simulink model "Microgrid_W"  (R2020a)
settings: Solver=ode15s  StartTime=0  StopTime=1440*1  MaxStep=1  RelTol=1e-3
libraries: simulink x4214, powerlib x685, simulink_extras x28, Microgrid_Library x18, powerlib_meascontrol x12
(part 29 of 48)

== system Microgrid_W/House 4 W1/Light 1/D2 ==
  Add : Sum
  Clock1 : Clock
  Constant : Constant
  Constant1 : Constant  Value=0
  Gain : Gain  Gain=t
  Interval Test : simulink/Logic and Bit Operations/Interval Test  IntervalClosedRight=on  uplimit=K_L1_Off_1+86400  IntervalClosedLeft=on  lowlimit=K_L1_On_1+86400  OutDataTypeStr=boolean
  Interval Test1 : simulink/Logic and Bit Operations/Interval Test  IntervalClosedRight=on  uplimit=K_L1_Off_2+86400  IntervalClosedLeft=on  lowlimit=K_L1_On_2+86400  OutDataTypeStr=boolean
  Switch : Switch  Criteria=u2 > Threshold  Threshold=0.5
  Switch1 : Switch  Criteria=u2 > Threshold  Threshold=0.5
  Out1 : Outport  VectorParamsAs1DForOutWhenUnconnected=off
  wires:
  Interval Test/1 -> Switch/2
  Switch/1 -> Add/1
  Interval Test1/1 -> Switch1/2
  Add/1 -> Out1/1
  Constant1/1 -> Switch/3, Switch1/3
  Constant/1 -> Switch/1, Switch1/1
  Switch1/1 -> Add/2
  Gain/1 -> Interval Test1/1, Interval Test/1
  Clock1/1 -> Gain/1

== system Microgrid_W/House 4 W1/Light 1/D3 ==
  Add : Sum
  Clock1 : Clock
  Constant : Constant
  Constant1 : Constant  Value=0
  Gain : Gain  Gain=t
  Interval Test : simulink/Logic and Bit Operations/Interval Test  IntervalClosedRight=on  uplimit=K_L1_Off_1+86400*2  IntervalClosedLeft=on  lowlimit=K_L1_On_1+86400*2  OutDataTypeStr=boolean
  Interval Test1 : simulink/Logic and Bit Operations/Interval Test  IntervalClosedRight=on  uplimit=K_L1_Off_2+86400*2  IntervalClosedLeft=on  lowlimit=K_L1_On_2+86400*2  OutDataTypeStr=boolean
  Switch : Switch  Criteria=u2 > Threshold  Threshold=0.5
  Switch1 : Switch  Criteria=u2 > Threshold  Threshold=0.5
  Out1 : Outport  VectorParamsAs1DForOutWhenUnconnected=off
  wires:
  Gain/1 -> Interval Test/1, Interval Test1/1
  Switch1/1 -> Add/2
  Constant/1 -> Switch1/1, Switch/1
  Constant1/1 -> Switch1/3, Switch/3
  Add/1 -> Out1/1
  Interval Test1/1 -> Switch1/2
  Switch/1 -> Add/1
  Interval Test/1 -> Switch/2
  Clock1/1 -> Gain/1

== system Microgrid_W/House 4 W1/Light 1/D4 ==
  Add : Sum
  Clock : Clock
  Constant : Constant
  Constant1 : Constant  Value=0
  Gain : Gain  Gain=t
  Interval Test : simulink/Logic and Bit Operations/Interval Test  IntervalClosedRight=on  uplimit=K_L1_Off_1+86400*3  IntervalClosedLeft=on  lowlimit=K_L1_On_1+86400*3  OutDataTypeStr=boolean
  Interval Test1 : simulink/Logic and Bit Operations/Interval Test  IntervalClosedRight=on  uplimit=K_L1_Off_2+86400*3  IntervalClosedLeft=on  lowlimit=K_L1_On_2+86400*3  OutDataTypeStr=boolean
  Switch : Switch  Criteria=u2 > Threshold  Threshold=0.5
  Switch1 : Switch  Criteria=u2 > Threshold  Threshold=0.5
  Out1 : Outport  VectorParamsAs1DForOutWhenUnconnected=off
  wires:
  Interval Test/1 -> Switch/2
  Switch/1 -> Add/1
  Interval Test1/1 -> Switch1/2
  Add/1 -> Out1/1
  Constant1/1 -> Switch/3, Switch1/3
  Constant/1 -> Switch/1, Switch1/1
  Switch1/1 -> Add/2
  Gain/1 -> Interval Test1/1, Interval Test/1
  Clock/1 -> Gain/1

== system Microgrid_W/House 4 W1/Light 1/D5 ==
  Add : Sum
  Clock : Clock
  Constant : Constant
  Constant1 : Constant  Value=0
  Gain : Gain  Gain=t
  Interval Test : simulink/Logic and Bit Operations/Interval Test  IntervalClosedRight=on  uplimit=K_L1_Off_1+86400*4  IntervalClosedLeft=on  lowlimit=K_L1_On_1+86400*4  OutDataTypeStr=boolean
  Interval Test1 : simulink/Logic and Bit Operations/Interval Test  IntervalClosedRight=on  uplimit=K_L1_Off_2+86400*4  IntervalClosedLeft=on  lowlimit=K_L1_On_2+86400*4  OutDataTypeStr=boolean
  Switch : Switch  Criteria=u2 > Threshold  Threshold=0.5
  Switch1 : Switch  Criteria=u2 > Threshold  Threshold=0.5
  Out1 : Outport  VectorParamsAs1DForOutWhenUnconnected=off
  wires:
  Gain/1 -> Interval Test/1, Interval Test1/1
  Switch1/1 -> Add/2
  Constant/1 -> Switch1/1, Switch/1
  Constant1/1 -> Switch1/3, Switch/3
  Add/1 -> Out1/1
  Interval Test1/1 -> Switch1/2
  Switch/1 -> Add/1
  Interval Test/1 -> Switch/2
  Clock/1 -> Gain/1

== system Microgrid_W/House 4 W1/Light 1/D6 ==
  Add : Sum
  Clock : Clock
  Constant : Constant
  Constant1 : Constant  Value=0
  Gain : Gain  Gain=t
  Interval Test : simulink/Logic and Bit Operations/Interval Test  IntervalClosedRight=on  uplimit=K_L1_Off_1+86400*5  IntervalClosedLeft=on  lowlimit=K_L1_On_1+86400*5  OutDataTypeStr=boolean
  Interval Test1 : simulink/Logic and Bit Operations/Interval Test  IntervalClosedRight=on  uplimit=K_L1_Off_2+86400*5  IntervalClosedLeft=on  lowlimit=K_L1_On_2+86400*5  OutDataTypeStr=boolean
  Switch : Switch  Criteria=u2 > Threshold  Threshold=0.5
  Switch1 : Switch  Criteria=u2 > Threshold  Threshold=0.5
  Out1 : Outport  VectorParamsAs1DForOutWhenUnconnected=off
  wires:
  Interval Test/1 -> Switch/2
  Switch/1 -> Add/1
  Interval Test1/1 -> Switch1/2
  Add/1 -> Out1/1
  Constant1/1 -> Switch/3, Switch1/3
  Constant/1 -> Switch/1, Switch1/1
  Switch1/1 -> Add/2
  Gain/1 -> Interval Test1/1, Interval Test/1
  Clock/1 -> Gain/1

== system Microgrid_W/House 4 W1/Light 1/D7 ==
  Add : Sum
  Clock : Clock
  Constant : Constant
  Constant1 : Constant  Value=0
  Gain : Gain  Gain=t
  Interval Test : simulink/Logic and Bit Operations/Interval Test  IntervalClosedRight=on  uplimit=K_L1_Off_1+86400*6  IntervalClosedLeft=on  lowlimit=K_L1_On_1+86400*6  OutDataTypeStr=boolean
  Interval Test1 : simulink/Logic and Bit Operations/Interval Test  IntervalClosedRight=on  uplimit=K_L1_Off_2+86400*6  IntervalClosedLeft=on  lowlimit=K_L1_On_2+86400*6  OutDataTypeStr=boolean
  Switch : Switch  Criteria=u2 > Threshold  Threshold=0.5
  Switch1 : Switch  Criteria=u2 > Threshold  Threshold=0.5
  Out1 : Outport  VectorParamsAs1DForOutWhenUnconnected=off
  wires:
  Gain/1 -> Interval Test/1, Interval Test1/1
  Switch1/1 -> Add/2
  Constant/1 -> Switch1/1, Switch/1
  Constant1/1 -> Switch1/3, Switch/3
  Add/1 -> Out1/1
  Interval Test1/1 -> Switch1/2
  Switch/1 -> Add/1
  Interval Test/1 -> Switch/2
  Clock/1 -> Gain/1

== system Microgrid_W/House 4 W1/Light 2/D1 ==
  Clock : Clock
  Constant : Constant
  Constant1 : Constant  Value=0
  Gain : Gain  Gain=t
  Interval Test : simulink/Logic and Bit Operations/Interval Test  IntervalClosedRight=on  uplimit=K_L2_Off_1  IntervalClosedLeft=on  lowlimit=K_L2_On_1  OutDataTypeStr=boolean
  Switch : Switch  Criteria=u2 > Threshold  Threshold=0.5
  Out1 : Outport  VectorParamsAs1DForOutWhenUnconnected=off
  wires:
  Interval Test/1 -> Switch/2
  Switch/1 -> Out1/1
  Constant1/1 -> Switch/3
  Constant/1 -> Switch/1
  Gain/1 -> Interval Test/1
  Clock/1 -> Gain/1

== system Microgrid_W/House 4 W1/Light 2/D2 ==
  Clock : Clock
  Constant : Constant
  Constant1 : Constant  Value=0
  Gain : Gain  Gain=t
  Interval Test : simulink/Logic and Bit Operations/Interval Test  IntervalClosedRight=on  uplimit=K_L2_Off_1+86400  IntervalClosedLeft=on  lowlimit=K_L2_On_1+86400  OutDataTypeStr=boolean
  Switch : Switch  Criteria=u2 > Threshold  Threshold=0.5
  Out1 : Outport  VectorParamsAs1DForOutWhenUnconnected=off
  wires:
  Gain/1 -> Interval Test/1
  Constant/1 -> Switch/1
  Constant1/1 -> Switch/3
  Switch/1 -> Out1/1
  Interval Test/1 -> Switch/2
  Clock/1 -> Gain/1

== system Microgrid_W/House 4 W1/Light 2/D3 ==
  Clock : Clock
  Constant : Constant
  Constant1 : Constant  Value=0
  Gain : Gain  Gain=t
  Interval Test : simulink/Logic and Bit Operations/Interval Test  IntervalClosedRight=on  uplimit=K_L2_Off_1+86400*2  IntervalClosedLeft=on  lowlimit=K_L2_On_1+86400*2  OutDataTypeStr=boolean
  Switch : Switch  Criteria=u2 > Threshold  Threshold=0.5
  Out1 : Outport  VectorParamsAs1DForOutWhenUnconnected=off
  wires:
  Interval Test/1 -> Switch/2
  Switch/1 -> Out1/1
  Constant1/1 -> Switch/3
  Constant/1 -> Switch/1
  Gain/1 -> Interval Test/1
  Clock/1 -> Gain/1

== system Microgrid_W/House 4 W1/Light 2/D4 ==
  Clock : Clock
  Constant : Constant
  Constant1 : Constant  Value=0
  Gain : Gain  Gain=t
  Interval Test : simulink/Logic and Bit Operations/Interval Test  IntervalClosedRight=on  uplimit=K_L2_Off_1+86400*3  IntervalClosedLeft=on  lowlimit=K_L2_On_1+86400*3  OutDataTypeStr=boolean
  Switch : Switch  Criteria=u2 > Threshold  Threshold=0.5
  Out1 : Outport  VectorParamsAs1DForOutWhenUnconnected=off
  wires:
  Gain/1 -> Interval Test/1
  Constant/1 -> Switch/1
  Constant1/1 -> Switch/3
  Switch/1 -> Out1/1
  Interval Test/1 -> Switch/2
  Clock/1 -> Gain/1

== system Microgrid_W/House 4 W1/Light 2/D5 ==
  Clock : Clock
  Constant : Constant
  Constant1 : Constant  Value=0
  Gain : Gain  Gain=t
  Interval Test : simulink/Logic and Bit Operations/Interval Test  IntervalClosedRight=on  uplimit=K_L2_Off_1+86400*4  IntervalClosedLeft=on  lowlimit=K_L2_On_1+86400*4  OutDataTypeStr=boolean
  Switch : Switch  Criteria=u2 > Threshold  Threshold=0.5
  Out1 : Outport  VectorParamsAs1DForOutWhenUnconnected=off
  wires:
  Interval Test/1 -> Switch/2
  Switch/1 -> Out1/1
  Constant1/1 -> Switch/3
  Constant/1 -> Switch/1
  Gain/1 -> Interval Test/1
  Clock/1 -> Gain/1

== system Microgrid_W/House 4 W1/Light 2/D6 ==
  Clock : Clock
  Constant : Constant
  Constant1 : Constant  Value=0
  Gain : Gain  Gain=t
  Interval Test : simulink/Logic and Bit Operations/Interval Test  IntervalClosedRight=on  uplimit=K_L2_Off_1+86400*5  IntervalClosedLeft=on  lowlimit=K_L2_On_1+86400*5  OutDataTypeStr=boolean
  Switch : Switch  Criteria=u2 > Threshold  Threshold=0.5
  Out1 : Outport  VectorParamsAs1DForOutWhenUnconnected=off
  wires:
  Gain/1 -> Interval Test/1
  Constant/1 -> Switch/1
  Constant1/1 -> Switch/3
  Switch/1 -> Out1/1
  Interval Test/1 -> Switch/2
  Clock/1 -> Gain/1

== system Microgrid_W/House 4 W1/Light 2/D7 ==
  Clock : Clock
  Constant : Constant
  Constant1 : Constant  Value=0
  Gain : Gain  Gain=t
  Interval Test : simulink/Logic and Bit Operations/Interval Test  IntervalClosedRight=on  uplimit=K_L2_Off_1+86400*6  IntervalClosedLeft=on  lowlimit=K_L2_On_1+86400*6  OutDataTypeStr=boolean
  Switch : Switch  Criteria=u2 > Threshold  Threshold=0.5
  Out1 : Outport  VectorParamsAs1DForOutWhenUnconnected=off
  wires:
  Interval Test/1 -> Switch/2
  Switch/1 -> Out1/1
  Constant1/1 -> Switch/3
  Constant/1 -> Switch/1
  Gain/1 -> Interval Test/1
  Clock/1 -> Gain/1

== system Microgrid_W/House 4 W1/Light 3/D1 ==
  Add : Sum
  Clock : Clock
  Constant : Constant
  Constant1 : Constant  Value=0
  Gain : Gain  Gain=t
  Interval Test : simulink/Logic and Bit Operations/Interval Test  IntervalClosedRight=on  uplimit=K_L3_Off_1  IntervalClosedLeft=on  lowlimit=K_L3_On_1  OutDataTypeStr=boolean
  Interval Test1 : simulink/Logic and Bit Operations/Interval Test  IntervalClosedRight=on  uplimit=K_L3_Off_2  IntervalClosedLeft=on  lowlimit=K_L3_On_2  OutDataTypeStr=boolean
  Switch : Switch  Criteria=u2 > Threshold  Threshold=0.5
  Switch1 : Switch  Criteria=u2 > Threshold  Threshold=0.5
  Out1 : Outport  VectorParamsAs1DForOutWhenUnconnected=off
  wires:
  Interval Test/1 -> Switch/2
  Switch/1 -> Add/1
  Interval Test1/1 -> Switch1/2
  Add/1 -> Out1/1
  Constant1/1 -> Switch/3, Switch1/3
  Constant/1 -> Switch/1, Switch1/1
  Switch1/1 -> Add/2
  Gain/1 -> Interval Test1/1, Interval Test/1
  Clock/1 -> Gain/1

== system Microgrid_W/House 4 W1/Light 3/D2 ==
  Add : Sum
  Clock : Clock
  Constant : Constant
  Constant1 : Constant  Value=0
  Gain : Gain  Gain=t
  Interval Test : simulink/Logic and Bit Operations/Interval Test  IntervalClosedRight=on  uplimit=K_L3_Off_1+86400  IntervalClosedLeft=on  lowlimit=K_L3_On_1+86400  OutDataTypeStr=boolean
  Interval Test1 : simulink/Logic and Bit Operations/Interval Test  IntervalClosedRight=on  uplimit=K_L3_Off_2+86400  IntervalClosedLeft=on  lowlimit=K_L3_On_2+86400  OutDataTypeStr=boolean
  Switch : Switch  Criteria=u2 > Threshold  Threshold=0.5
  Switch1 : Switch  Criteria=u2 > Threshold  Threshold=0.5
  Out1 : Outport  VectorParamsAs1DForOutWhenUnconnected=off
  wires:
  Gain/1 -> Interval Test/1, Interval Test1/1
  Switch1/1 -> Add/2
  Constant/1 -> Switch1/1, Switch/1
  Constant1/1 -> Switch1/3, Switch/3
  Add/1 -> Out1/1
  Interval Test1/1 -> Switch1/2
  Switch/1 -> Add/1
  Interval Test/1 -> Switch/2
  Clock/1 -> Gain/1

== system Microgrid_W/House 4 W1/Light 3/D3 ==
  Add : Sum
  Clock : Clock
  Constant : Constant
  Constant1 : Constant  Value=0
  Gain : Gain  Gain=t
  Interval Test : simulink/Logic and Bit Operations/Interval Test  IntervalClosedRight=on  uplimit=K_L3_Off_1+86400*2  IntervalClosedLeft=on  lowlimit=K_L3_On_1+86400*2  OutDataTypeStr=boolean
  Interval Test1 : simulink/Logic and Bit Operations/Interval Test  IntervalClosedRight=on  uplimit=K_L3_Off_2+86400*2  IntervalClosedLeft=on  lowlimit=K_L3_On_2+86400*2  OutDataTypeStr=boolean
  Switch : Switch  Criteria=u2 > Threshold  Threshold=0.5
  Switch1 : Switch  Criteria=u2 > Threshold  Threshold=0.5
  Out1 : Outport  VectorParamsAs1DForOutWhenUnconnected=off
  wires:
  Interval Test/1 -> Switch/2
  Switch/1 -> Add/1
  Interval Test1/1 -> Switch1/2
  Add/1 -> Out1/1
  Constant1/1 -> Switch/3, Switch1/3
  Constant/1 -> Switch/1, Switch1/1
  Switch1/1 -> Add/2
  Gain/1 -> Interval Test1/1, Interval Test/1
  Clock/1 -> Gain/1

== system Microgrid_W/House 4 W1/Light 3/D4 ==
  Add : Sum
  Clock : Clock
  Constant : Constant
  Constant1 : Constant  Value=0
  Gain : Gain  Gain=t
  Interval Test : simulink/Logic and Bit Operations/Interval Test  IntervalClosedRight=on  uplimit=K_L3_Off_1+86400*3  IntervalClosedLeft=on  lowlimit=K_L3_On_1+86400*3  OutDataTypeStr=boolean
  Interval Test1 : simulink/Logic and Bit Operations/Interval Test  IntervalClosedRight=on  uplimit=K_L3_Off_2+86400*3  IntervalClosedLeft=on  lowlimit=K_L3_On_2+86400*3  OutDataTypeStr=boolean
  Switch : Switch  Criteria=u2 > Threshold  Threshold=0.5
  Switch1 : Switch  Criteria=u2 > Threshold  Threshold=0.5
  Out1 : Outport  VectorParamsAs1DForOutWhenUnconnected=off
  wires:
  Gain/1 -> Interval Test/1, Interval Test1/1
  Switch1/1 -> Add/2
  Constant/1 -> Switch1/1, Switch/1
  Constant1/1 -> Switch1/3, Switch/3
  Add/1 -> Out1/1
  Interval Test1/1 -> Switch1/2
  Switch/1 -> Add/1
  Interval Test/1 -> Switch/2
  Clock/1 -> Gain/1

== system Microgrid_W/House 4 W1/Light 3/D5 ==
  Add : Sum
  Clock : Clock
  Constant : Constant
  Constant1 : Constant  Value=0
  Gain : Gain  Gain=t
  Interval Test : simulink/Logic and Bit Operations/Interval Test  IntervalClosedRight=on  uplimit=K_L3_Off_1+86400*4  IntervalClosedLeft=on  lowlimit=K_L3_On_1+86400*4  OutDataTypeStr=boolean
  Interval Test1 : simulink/Logic and Bit Operations/Interval Test  IntervalClosedRight=on  uplimit=K_L3_Off_2+86400*4  IntervalClosedLeft=on  lowlimit=K_L3_On_2+86400*4  OutDataTypeStr=boolean
  Switch : Switch  Criteria=u2 > Threshold  Threshold=0.5
  Switch1 : Switch  Criteria=u2 > Threshold  Threshold=0.5
  Out1 : Outport  VectorParamsAs1DForOutWhenUnconnected=off
  wires:
  Interval Test/1 -> Switch/2
  Switch/1 -> Add/1
  Interval Test1/1 -> Switch1/2
  Add/1 -> Out1/1
  Constant1/1 -> Switch/3, Switch1/3
  Constant/1 -> Switch/1, Switch1/1
  Switch1/1 -> Add/2
  Gain/1 -> Interval Test1/1, Interval Test/1
  Clock/1 -> Gain/1

== system Microgrid_W/House 4 W1/Light 3/D6 ==
  Add : Sum
  Clock : Clock
  Constant : Constant
  Constant1 : Constant  Value=0
  Gain : Gain  Gain=t
  Interval Test : simulink/Logic and Bit Operations/Interval Test  IntervalClosedRight=on  uplimit=K_L3_Off_1+86400*5  IntervalClosedLeft=on  lowlimit=K_L3_On_1+86400*5  OutDataTypeStr=boolean
  Interval Test1 : simulink/Logic and Bit Operations/Interval Test  IntervalClosedRight=on  uplimit=K_L3_Off_2+86400*5  IntervalClosedLeft=on  lowlimit=K_L3_On_2+86400*5  OutDataTypeStr=boolean
  Switch : Switch  Criteria=u2 > Threshold  Threshold=0.5
  Switch1 : Switch  Criteria=u2 > Threshold  Threshold=0.5
  Out1 : Outport  VectorParamsAs1DForOutWhenUnconnected=off
  wires:
  ? -> Interval Test/1, Interval Test1/1
  Switch1/1 -> Add/2
  Constant/1 -> Switch1/1, Switch/1
  Constant1/1 -> Switch1/3, Switch/3
  Add/1 -> Out1/1
  Interval Test1/1 -> Switch1/2
  Switch/1 -> Add/1
  Interval Test/1 -> Switch/2
  Clock/1 -> Gain/1

== system Microgrid_W/House 4 W1/Light 3/D7 ==
  Add : Sum
  Clock : Clock
  Constant : Constant
  Constant1 : Constant  Value=0
  Gain : Gain  Gain=t
  Interval Test : simulink/Logic and Bit Operations/Interval Test  IntervalClosedRight=on  uplimit=K_L3_Off_1+86400*6  IntervalClosedLeft=on  lowlimit=K_L3_On_1+86400*6  OutDataTypeStr=boolean
  Interval Test1 : simulink/Logic and Bit Operations/Interval Test  IntervalClosedRight=on  uplimit=K_L3_Off_2+86400*6  IntervalClosedLeft=on  lowlimit=K_L3_On_2+86400*6  OutDataTypeStr=boolean
  Switch : Switch  Criteria=u2 > Threshold  Threshold=0.5
  Switch1 : Switch  Criteria=u2 > Threshold  Threshold=0.5
  Out1 : Outport  VectorParamsAs1DForOutWhenUnconnected=off
  wires:
  Interval Test/1 -> Switch/2
  Switch/1 -> Add/1
  Interval Test1/1 -> Switch1/2
  Add/1 -> Out1/1
  Constant1/1 -> Switch/3, Switch1/3
  Constant/1 -> Switch/1, Switch1/1
  Switch1/1 -> Add/2
  Gain/1 -> Interval Test1/1, Interval Test/1
  Clock/1 -> Gain/1

== system Microgrid_W/House 4 W1/Light 4/D1 ==
  Clock : Clock
  Constant : Constant
  Constant1 : Constant  Value=0
  Gain : Gain  Gain=t
  Interval Test : simulink/Logic and Bit Operations/Interval Test  IntervalClosedRight=on  uplimit=K_L4_Off_1  IntervalClosedLeft=on  lowlimit=K_L4_On_1  OutDataTypeStr=boolean
  Switch : Switch  Criteria=u2 > Threshold  Threshold=0.5
  Out1 : Outport  VectorParamsAs1DForOutWhenUnconnected=off
  wires:
  Interval Test/1 -> Switch/2
  Switch/1 -> Out1/1
  Constant1/1 -> Switch/3
  Constant/1 -> Switch/1
  Gain/1 -> Interval Test/1
  Clock/1 -> Gain/1

== system Microgrid_W/House 4 W1/Light 4/D2 ==
  Clock : Clock
  Constant : Constant
  Constant1 : Constant  Value=0
  Gain : Gain  Gain=t
  Interval Test : simulink/Logic and Bit Operations/Interval Test  IntervalClosedRight=on  uplimit=K_L4_Off_1+86400  IntervalClosedLeft=on  lowlimit=K_L4_On_1+86400  OutDataTypeStr=boolean
  Switch : Switch  Criteria=u2 > Threshold  Threshold=0.5
  Out1 : Outport  VectorParamsAs1DForOutWhenUnconnected=off
  wires:
  Gain/1 -> Interval Test/1
  Constant/1 -> Switch/1
  Constant1/1 -> Switch/3
  Switch/1 -> Out1/1
  Interval Test/1 -> Switch/2
  Clock/1 -> Gain/1

== system Microgrid_W/House 4 W1/Light 4/D3 ==
  Clock : Clock
  Constant : Constant
  Constant1 : Constant  Value=0
  Gain : Gain  Gain=t
  Interval Test : simulink/Logic and Bit Operations/Interval Test  IntervalClosedRight=on  uplimit=K_L4_Off_1+86400*2  IntervalClosedLeft=on  lowlimit=K_L4_On_1+86400*2  OutDataTypeStr=boolean
  Switch : Switch  Criteria=u2 > Threshold  Threshold=0.5
  Out1 : Outport  VectorParamsAs1DForOutWhenUnconnected=off
  wires:
  Interval Test/1 -> Switch/2
  Switch/1 -> Out1/1
  Constant1/1 -> Switch/3
  Constant/1 -> Switch/1
  Gain/1 -> Interval Test/1
  Clock/1 -> Gain/1

== system Microgrid_W/House 4 W1/Light 4/D4 ==
  Clock : Clock
  Constant : Constant
  Constant1 : Constant  Value=0
  Gain : Gain  Gain=t
  Interval Test : simulink/Logic and Bit Operations/Interval Test  IntervalClosedRight=on  uplimit=K_L4_Off_1+86400*3  IntervalClosedLeft=on  lowlimit=K_L4_On_1+86400*3  OutDataTypeStr=boolean
  Switch : Switch  Criteria=u2 > Threshold  Threshold=0.5
  Out1 : Outport  VectorParamsAs1DForOutWhenUnconnected=off
  wires:
  Gain/1 -> Interval Test/1
  Constant/1 -> Switch/1
  Constant1/1 -> Switch/3
  Switch/1 -> Out1/1
  Interval Test/1 -> Switch/2
  Clock/1 -> Gain/1

== system Microgrid_W/House 4 W1/Light 4/D5 ==
  Clock : Clock
  Constant : Constant
  Constant1 : Constant  Value=0
  Gain : Gain  Gain=t
  Interval Test : simulink/Logic and Bit Operations/Interval Test  IntervalClosedRight=on  uplimit=K_L4_Off_1+86400*4  IntervalClosedLeft=on  lowlimit=K_L4_On_1+86400*4  OutDataTypeStr=boolean
  Switch : Switch  Criteria=u2 > Threshold  Threshold=0.5
  Out1 : Outport  VectorParamsAs1DForOutWhenUnconnected=off
  wires:
  Interval Test/1 -> Switch/2
  Switch/1 -> Out1/1
  Constant1/1 -> Switch/3
  Constant/1 -> Switch/1
  Gain/1 -> Interval Test/1
  Clock/1 -> Gain/1

== system Microgrid_W/House 4 W1/Light 4/D6 ==
  Clock : Clock
  Constant : Constant
  Constant1 : Constant  Value=0
  Gain : Gain  Gain=t
  Interval Test : simulink/Logic and Bit Operations/Interval Test  IntervalClosedRight=on  uplimit=K_L4_Off_1+86400*5  IntervalClosedLeft=on  lowlimit=K_L4_On_1+86400*5  OutDataTypeStr=boolean
  Switch : Switch  Criteria=u2 > Threshold  Threshold=0.5
  Out1 : Outport  VectorParamsAs1DForOutWhenUnconnected=off
  wires:
  Gain/1 -> Interval Test/1
  Constant/1 -> Switch/1
  Constant1/1 -> Switch/3
  Switch/1 -> Out1/1
  Interval Test/1 -> Switch/2
  Clock/1 -> Gain/1

== system Microgrid_W/House 4 W1/Light 4/D7 ==
  Clock : Clock
  Constant : Constant
  Constant1 : Constant  Value=0
  Gain : Gain  Gain=t
  Interval Test : simulink/Logic and Bit Operations/Interval Test  IntervalClosedRight=on  uplimit=K_L4_Off_1+86400*6  IntervalClosedLeft=on  lowlimit=K_L4_On_1+86400*6  OutDataTypeStr=boolean
  Switch : Switch  Criteria=u2 > Threshold  Threshold=0.5
  Out1 : Outport  VectorParamsAs1DForOutWhenUnconnected=off
  wires:
  Interval Test/1 -> Switch/2
  Switch/1 -> Out1/1
  Constant1/1 -> Switch/3
  Constant/1 -> Switch/1
  Gain/1 -> Interval Test/1
  Clock/1 -> Gain/1

== system Microgrid_W/House 4 W1/Light 5/D1 ==
  Add : Sum
  Clock : Clock
  Constant : Constant
  Constant1 : Constant  Value=0
  Gain : Gain  Gain=t
  Interval Test : simulink/Logic and Bit Operations/Interval Test  IntervalClosedRight=on  uplimit=K_L5_Off_1  IntervalClosedLeft=on  lowlimit=K_L5_On_1  OutDataTypeStr=boolean
  Interval Test1 : simulink/Logic and Bit Operations/Interval Test  IntervalClosedRight=on  uplimit=K_L5_Off_2  IntervalClosedLeft=on  lowlimit=K_L5_On_2  OutDataTypeStr=boolean
  Switch : Switch  Criteria=u2 > Threshold  Threshold=0.5
  Switch1 : Switch  Criteria=u2 > Threshold  Threshold=0.5
  Out1 : Outport  VectorParamsAs1DForOutWhenUnconnected=off
  wires:
  Gain/1 -> Interval Test/1, Interval Test1/1
  Switch1/1 -> Add/2
  Constant/1 -> Switch1/1, Switch/1
  Constant1/1 -> Switch1/3, Switch/3
  Add/1 -> Out1/1
  Interval Test1/1 -> Switch1/2
  Switch/1 -> Add/1
  Interval Test/1 -> Switch/2
  Clock/1 -> Gain/1

== system Microgrid_W/House 4 W1/Light 5/D2 ==
  Add : Sum
  Clock : Clock
  Constant : Constant
  Constant1 : Constant  Value=0
  Gain : Gain  Gain=t
  Interval Test : simulink/Logic and Bit Operations/Interval Test  IntervalClosedRight=on  uplimit=K_L5_Off_1+86400  IntervalClosedLeft=on  lowlimit=K_L5_On_1+86400  OutDataTypeStr=boolean
  Interval Test1 : simulink/Logic and Bit Operations/Interval Test  IntervalClosedRight=on  uplimit=K_L5_Off_2+86400  IntervalClosedLeft=on  lowlimit=K_L5_On_2+86400  OutDataTypeStr=boolean
  Switch : Switch  Criteria=u2 > Threshold  Threshold=0.5
  Switch1 : Switch  Criteria=u2 > Threshold  Threshold=0.5
  Out1 : Outport  VectorParamsAs1DForOutWhenUnconnected=off
  wires:
  Interval Test/1 -> Switch/2
  Switch/1 -> Add/1
  Interval Test1/1 -> Switch1/2
  Add/1 -> Out1/1
  Constant1/1 -> Switch/3, Switch1/3
  Constant/1 -> Switch/1, Switch1/1
  Switch1/1 -> Add/2
  Gain/1 -> Interval Test1/1, Interval Test/1
  Clock/1 -> Gain/1

== system Microgrid_W/House 4 W1/Light 5/D3 ==
  Add : Sum
  Clock : Clock
  Constant : Constant
  Constant1 : Constant  Value=0
  Gain : Gain  Gain=t
  Interval Test : simulink/Logic and Bit Operations/Interval Test  IntervalClosedRight=on  uplimit=K_L5_Off_1+86400*2  IntervalClosedLeft=on  lowlimit=K_L5_On_1+86400*2  OutDataTypeStr=boolean
  Interval Test1 : simulink/Logic and Bit Operations/Interval Test  IntervalClosedRight=on  uplimit=K_L5_Off_2+86400*2  IntervalClosedLeft=on  lowlimit=K_L5_On_2+86400*2  OutDataTypeStr=boolean
  Switch : Switch  Criteria=u2 > Threshold  Threshold=0.5
  Switch1 : Switch  Criteria=u2 > Threshold  Threshold=0.5
  Out1 : Outport  VectorParamsAs1DForOutWhenUnconnected=off
  wires:
  Gain/1 -> Interval Test/1, Interval Test1/1
  Switch1/1 -> Add/2
  Constant/1 -> Switch1/1, Switch/1
  Constant1/1 -> Switch1/3, Switch/3
  Add/1 -> Out1/1
  Interval Test1/1 -> Switch1/2
  Switch/1 -> Add/1
  Interval Test/1 -> Switch/2
  Clock/1 -> Gain/1

== system Microgrid_W/House 4 W1/Light 5/D4 ==
  Add : Sum
  Clock : Clock
  Constant : Constant
  Constant1 : Constant  Value=0
  Gain : Gain  Gain=t
  Interval Test : simulink/Logic and Bit Operations/Interval Test  IntervalClosedRight=on  uplimit=K_L5_Off_1+86400*3  IntervalClosedLeft=on  lowlimit=K_L5_On_1+86400*3  OutDataTypeStr=boolean
  Interval Test1 : simulink/Logic and Bit Operations/Interval Test  IntervalClosedRight=on  uplimit=K_L5_Off_2+86400*3  IntervalClosedLeft=on  lowlimit=K_L5_On_2+86400*3  OutDataTypeStr=boolean
  Switch : Switch  Criteria=u2 > Threshold  Threshold=0.5
  Switch1 : Switch  Criteria=u2 > Threshold  Threshold=0.5
  Out1 : Outport  VectorParamsAs1DForOutWhenUnconnected=off
  wires:
  Interval Test/1 -> Switch/2
  Switch/1 -> Add/1
  Interval Test1/1 -> Switch1/2
  Add/1 -> Out1/1
  Constant1/1 -> Switch/3, Switch1/3
  Constant/1 -> Switch/1, Switch1/1
  Switch1/1 -> Add/2
  Gain/1 -> Interval Test1/1, Interval Test/1
  Clock/1 -> Gain/1

== system Microgrid_W/House 4 W1/Light 5/D5 ==
  Add : Sum
  Clock : Clock
  Constant : Constant
  Constant1 : Constant  Value=0
  Gain : Gain  Gain=t
  Interval Test : simulink/Logic and Bit Operations/Interval Test  IntervalClosedRight=on  uplimit=K_L5_Off_1+86400*4  IntervalClosedLeft=on  lowlimit=K_L5_On_1+86400*4  OutDataTypeStr=boolean
  Interval Test1 : simulink/Logic and Bit Operations/Interval Test  IntervalClosedRight=on  uplimit=K_L5_Off_2+86400*4  IntervalClosedLeft=on  lowlimit=K_L5_On_2+86400*4  OutDataTypeStr=boolean
  Switch : Switch  Criteria=u2 > Threshold  Threshold=0.5
  Switch1 : Switch  Criteria=u2 > Threshold  Threshold=0.5
  Out1 : Outport  VectorParamsAs1DForOutWhenUnconnected=off
  wires:
  Gain/1 -> Interval Test/1, Interval Test1/1
  Switch1/1 -> Add/2
  Constant/1 -> Switch1/1, Switch/1
  Constant1/1 -> Switch1/3, Switch/3
  Add/1 -> Out1/1
  Interval Test1/1 -> Switch1/2
  Switch/1 -> Add/1
  Interval Test/1 -> Switch/2
  Clock/1 -> Gain/1

== system Microgrid_W/House 4 W1/Light 5/D6 ==
  Add : Sum
  Clock : Clock
  Constant : Constant
  Constant1 : Constant  Value=0
  Gain : Gain  Gain=t
  Interval Test : simulink/Logic and Bit Operations/Interval Test  IntervalClosedRight=on  uplimit=K_L5_Off_1+86400*5  IntervalClosedLeft=on  lowlimit=K_L5_On_1+86400*5  OutDataTypeStr=boolean
  Interval Test1 : simulink/Logic and Bit Operations/Interval Test  IntervalClosedRight=on  uplimit=K_L5_Off_2+86400*5  IntervalClosedLeft=on  lowlimit=K_L5_On_2+86400*5  OutDataTypeStr=boolean
  Switch : Switch  Criteria=u2 > Threshold  Threshold=0.5
  Switch1 : Switch  Criteria=u2 > Threshold  Threshold=0.5
  Out1 : Outport  VectorParamsAs1DForOutWhenUnconnected=off
  wires:
  Interval Test/1 -> Switch/2
  Switch/1 -> Add/1
  Interval Test1/1 -> Switch1/2
  Add/1 -> Out1/1
  Constant1/1 -> Switch/3, Switch1/3
  Constant/1 -> Switch/1, Switch1/1
  Switch1/1 -> Add/2
  Gain/1 -> Interval Test1/1, Interval Test/1
  Clock/1 -> Gain/1

== system Microgrid_W/House 4 W1/Light 5/D7 ==
  Add : Sum
  Clock : Clock
  Constant : Constant
  Constant1 : Constant  Value=0
  Gain : Gain  Gain=t
  Interval Test : simulink/Logic and Bit Operations/Interval Test  IntervalClosedRight=on  uplimit=K_L5_Off_1+86400*6  IntervalClosedLeft=on  lowlimit=K_L5_On_1+86400*6  OutDataTypeStr=boolean
  Interval Test1 : simulink/Logic and Bit Operations/Interval Test  IntervalClosedRight=on  uplimit=K_L5_Off_2+86400*6  IntervalClosedLeft=on  lowlimit=K_L5_On_2+86400*6  OutDataTypeStr=boolean
  Switch : Switch  Criteria=u2 > Threshold  Threshold=0.5
  Switch1 : Switch  Criteria=u2 > Threshold  Threshold=0.5
  Out1 : Outport  VectorParamsAs1DForOutWhenUnconnected=off
  wires:
  Gain/1 -> Interval Test/1, Interval Test1/1
  Switch1/1 -> Add/2
  Constant/1 -> Switch1/1, Switch/1
  Constant1/1 -> Switch1/3, Switch/3
  Add/1 -> Out1/1
  Interval Test1/1 -> Switch1/2
  Switch/1 -> Add/1
  Interval Test/1 -> Switch/2
  Clock/1 -> Gain/1

== system Microgrid_W/House 4 W1/Light 6/D1 ==
  Clock : Clock
  Constant : Constant
  Constant1 : Constant  Value=0
  Gain : Gain  Gain=t
  Interval Test : simulink/Logic and Bit Operations/Interval Test  IntervalClosedRight=on  uplimit=K_L6_Off_1  IntervalClosedLeft=on  lowlimit=K_L6_On_1  OutDataTypeStr=boolean
  Switch : Switch  Criteria=u2 > Threshold  Threshold=0.5
  Out1 : Outport  VectorParamsAs1DForOutWhenUnconnected=off
  wires:
  Interval Test/1 -> Switch/2
  Switch/1 -> Out1/1
  Constant1/1 -> Switch/3
  Constant/1 -> Switch/1
  Gain/1 -> Interval Test/1
  Clock/1 -> Gain/1

== system Microgrid_W/House 4 W1/Light 6/D2 ==
  Clock : Clock
  Constant : Constant
  Constant1 : Constant  Value=0
  Gain : Gain  Gain=t
  Interval Test : simulink/Logic and Bit Operations/Interval Test  IntervalClosedRight=on  uplimit=K_L6_Off_1+86400  IntervalClosedLeft=on  lowlimit=K_L6_On_1+86400  OutDataTypeStr=boolean
  Switch : Switch  Criteria=u2 > Threshold  Threshold=0.5
  Out1 : Outport  VectorParamsAs1DForOutWhenUnconnected=off
  wires:
  Gain/1 -> Interval Test/1
  Constant/1 -> Switch/1
  Constant1/1 -> Switch/3
  Switch/1 -> Out1/1
  Interval Test/1 -> Switch/2
  Clock/1 -> Gain/1

== system Microgrid_W/House 4 W1/Light 6/D3 ==
  Clock : Clock
  Constant : Constant
  Constant1 : Constant  Value=0
  Gain : Gain  Gain=t
  Interval Test : simulink/Logic and Bit Operations/Interval Test  IntervalClosedRight=on  uplimit=K_L6_Off_1+86400*2  IntervalClosedLeft=on  lowlimit=K_L6_On_1+86400*2  OutDataTypeStr=boolean
  Switch : Switch  Criteria=u2 > Threshold  Threshold=0.5
  Out1 : Outport  VectorParamsAs1DForOutWhenUnconnected=off
  wires:
  Interval Test/1 -> Switch/2
  Switch/1 -> Out1/1
  Constant1/1 -> Switch/3
  Constant/1 -> Switch/1
  Gain/1 -> Interval Test/1
  Clock/1 -> Gain/1

== system Microgrid_W/House 4 W1/Light 6/D4 ==
  Clock : Clock
  Constant : Constant
  Constant1 : Constant  Value=0
  Gain : Gain  Gain=t
  Interval Test : simulink/Logic and Bit Operations/Interval Test  IntervalClosedRight=on  uplimit=K_L6_Off_1+86400*3  IntervalClosedLeft=on  lowlimit=K_L6_On_1+86400*3  OutDataTypeStr=boolean
  Switch : Switch  Criteria=u2 > Threshold  Threshold=0.5
  Out1 : Outport  VectorParamsAs1DForOutWhenUnconnected=off
  wires:
  Gain/1 -> Interval Test/1
  Constant/1 -> Switch/1
  Constant1/1 -> Switch/3
  Switch/1 -> Out1/1
  Interval Test/1 -> Switch/2
  Clock/1 -> Gain/1

== system Microgrid_W/House 4 W1/Light 6/D5 ==
  Clock : Clock
  Constant : Constant
  Constant1 : Constant  Value=0
  Gain : Gain  Gain=t
  Interval Test : simulink/Logic and Bit Operations/Interval Test  IntervalClosedRight=on  uplimit=K_L6_Off_1+86400*4  IntervalClosedLeft=on  lowlimit=K_L6_On_1+86400*4  OutDataTypeStr=boolean
  Switch : Switch  Criteria=u2 > Threshold  Threshold=0.5
  Out1 : Outport  VectorParamsAs1DForOutWhenUnconnected=off
  wires:
  Interval Test/1 -> Switch/2
  Switch/1 -> Out1/1
  Constant1/1 -> Switch/3
  Constant/1 -> Switch/1
  Gain/1 -> Interval Test/1
  Clock/1 -> Gain/1

== system Microgrid_W/House 4 W1/Light 6/D6 ==
  Clock : Clock
  Constant : Constant
  Constant1 : Constant  Value=0
  Gain : Gain  Gain=t
  Interval Test : simulink/Logic and Bit Operations/Interval Test  IntervalClosedRight=on  uplimit=K_L6_Off_1+86400*5  IntervalClosedLeft=on  lowlimit=K_L6_On_1+86400*5  OutDataTypeStr=boolean
  Switch : Switch  Criteria=u2 > Threshold  Threshold=0.5
  Out1 : Outport  VectorParamsAs1DForOutWhenUnconnected=off
  wires:
  Gain/1 -> Interval Test/1
  Constant/1 -> Switch/1
  Constant1/1 -> Switch/3
  Switch/1 -> Out1/1
  Interval Test/1 -> Switch/2
  Clock/1 -> Gain/1

== system Microgrid_W/House 4 W1/Light 6/D7 ==
  Clock : Clock
  Constant : Constant
  Constant1 : Constant  Value=0
  Gain : Gain  Gain=t
  Interval Test : simulink/Logic and Bit Operations/Interval Test  IntervalClosedRight=on  uplimit=K_L6_Off_1+86400*6  IntervalClosedLeft=on  lowlimit=K_L6_On_1+86400*6  OutDataTypeStr=boolean
  Switch : Switch  Criteria=u2 > Threshold  Threshold=0.5
  Out1 : Outport  VectorParamsAs1DForOutWhenUnconnected=off
  wires:
  Interval Test/1 -> Switch/2
  Switch/1 -> Out1/1
  Constant1/1 -> Switch/3
  Constant/1 -> Switch/1
  Gain/1 -> Interval Test/1
  Clock/1 -> Gain/1

== system Microgrid_W/House 4 W1/Oven/D1 ==
  Clock : Clock
  Constant : Constant
  Constant1 : Constant  Value=0
  Gain : Gain  Gain=t
  Interval Test : simulink/Logic and Bit Operations/Interval Test  IntervalClosedRight=on  uplimit=Oven_Off_1  IntervalClosedLeft=on  lowlimit=Oven_On_1  OutDataTypeStr=boolean
  Switch : Switch  Criteria=u2 > Threshold  Threshold=0.5
  Out1 : Outport  VectorParamsAs1DForOutWhenUnconnected=off
  wires:
  Interval Test/1 -> Switch/2
  Switch/1 -> Out1/1
  Constant1/1 -> Switch/3
  Constant/1 -> Switch/1
  Gain/1 -> Interval Test/1
  Clock/1 -> Gain/1

== system Microgrid_W/House 4 W1/Oven/D2 ==
  Clock : Clock
  Constant : Constant
  Constant1 : Constant  Value=0
  Gain : Gain  Gain=t
  Interval Test : simulink/Logic and Bit Operations/Interval Test  IntervalClosedRight=on  uplimit=Oven_Off_1+86400  IntervalClosedLeft=on  lowlimit=Oven_On_1+86400  OutDataTypeStr=boolean
  Switch : Switch  Criteria=u2 > Threshold  Threshold=0.5
  Out1 : Outport  VectorParamsAs1DForOutWhenUnconnected=off
  wires:
  Gain/1 -> Interval Test/1
  Constant/1 -> Switch/1
  Constant1/1 -> Switch/3
  Switch/1 -> Out1/1
  Interval Test/1 -> Switch/2
  Clock/1 -> Gain/1

== system Microgrid_W/House 4 W1/Oven/D3 ==
  Clock : Clock
  Constant : Constant
  Constant1 : Constant  Value=0
  Gain : Gain  Gain=t
  Interval Test : simulink/Logic and Bit Operations/Interval Test  IntervalClosedRight=on  uplimit=Oven_Off_1+86400*2  IntervalClosedLeft=on  lowlimit=Oven_On_1+86400*2  OutDataTypeStr=boolean
  Switch : Switch  Criteria=u2 > Threshold  Threshold=0.5
  Out1 : Outport  VectorParamsAs1DForOutWhenUnconnected=off
  wires:
  Interval Test/1 -> Switch/2
  Switch/1 -> Out1/1
  Constant1/1 -> Switch/3
  Constant/1 -> Switch/1
  Gain/1 -> Interval Test/1
  Clock/1 -> Gain/1

== system Microgrid_W/House 4 W1/Oven/D4 ==
  Clock : Clock
  Constant : Constant
  Constant1 : Constant  Value=0
  Gain : Gain  Gain=t
  Interval Test : simulink/Logic and Bit Operations/Interval Test  IntervalClosedRight=on  uplimit=Oven_Off_1+86400*3  IntervalClosedLeft=on  lowlimit=Oven_On_1+86400*3  OutDataTypeStr=boolean
  Switch : Switch  Criteria=u2 > Threshold  Threshold=0.5
  Out1 : Outport  VectorParamsAs1DForOutWhenUnconnected=off
  wires:
  Gain/1 -> Interval Test/1
  Constant/1 -> Switch/1
  Constant1/1 -> Switch/3
  Switch/1 -> Out1/1
  Interval Test/1 -> Switch/2
  Clock/1 -> Gain/1

== system Microgrid_W/House 4 W1/Oven/D5 ==
  Clock : Clock
  Constant : Constant
  Constant1 : Constant  Value=0
  Gain : Gain  Gain=t
  Interval Test : simulink/Logic and Bit Operations/Interval Test  IntervalClosedRight=on  uplimit=Oven_Off_1+86400*4  IntervalClosedLeft=on  lowlimit=Oven_On_1+86400*4  OutDataTypeStr=boolean
  Switch : Switch  Criteria=u2 > Threshold  Threshold=0.5
  Out1 : Outport  VectorParamsAs1DForOutWhenUnconnected=off
  wires:
  Interval Test/1 -> Switch/2
  Switch/1 -> Out1/1
  Constant1/1 -> Switch/3
  Constant/1 -> Switch/1
  Gain/1 -> Interval Test/1
  Clock/1 -> Gain/1

== system Microgrid_W/House 4 W1/Oven/D6 ==
  Clock : Clock
  Constant : Constant
  Constant1 : Constant  Value=0
  Gain : Gain  Gain=t
  Interval Test : simulink/Logic and Bit Operations/Interval Test  IntervalClosedRight=on  uplimit=Oven_Off_1+86400*5  IntervalClosedLeft=on  lowlimit=Oven_On_1+86400*5  OutDataTypeStr=boolean
  Switch : Switch  Criteria=u2 > Threshold  Threshold=0.5
  Out1 : Outport  VectorParamsAs1DForOutWhenUnconnected=off
  wires:
  Gain/1 -> Interval Test/1
  Constant/1 -> Switch/1
  Constant1/1 -> Switch/3
  Switch/1 -> Out1/1
  Interval Test/1 -> Switch/2
  Clock/1 -> Gain/1

== system Microgrid_W/House 4 W1/Oven/D7 ==
  Clock : Clock
  Constant : Constant
  Constant1 : Constant  Value=0
  Gain : Gain  Gain=t
  Interval Test : simulink/Logic and Bit Operations/Interval Test  IntervalClosedRight=on  uplimit=Oven_Off_1+86400*6  IntervalClosedLeft=on  lowlimit=Oven_On_1+86400*6  OutDataTypeStr=boolean
  Switch : Switch  Criteria=u2 > Threshold  Threshold=0.5
  Out1 : Outport  VectorParamsAs1DForOutWhenUnconnected=off
  wires:
  Interval Test/1 -> Switch/2
  Switch/1 -> Out1/1
  Constant1/1 -> Switch/3
  Constant/1 -> Switch/1
  Gain/1 -> Interval Test/1
  Clock/1 -> Gain/1

== system Microgrid_W/House 4 W1/Phone_Charger/D1 ==
  Add : Sum
  Clock : Clock
  Constant : Constant
  Constant1 : Constant  Value=0
  Gain : Gain  Gain=t
  Interval Test : simulink/Logic and Bit Operations/Interval Test  IntervalClosedRight=on  uplimit=Phone_C_1_Off_a  IntervalClosedLeft=on  lowlimit=Phone_C_1_On_a  OutDataTypeStr=boolean
  Interval Test1 : simulink/Logic and Bit Operations/Interval Test  IntervalClosedRight=on  uplimit=Phone_C_1_Off_b  IntervalClosedLeft=on  lowlimit=Phone_C_1_On_b  OutDataTypeStr=boolean
  Switch : Switch  Criteria=u2 > Threshold  Threshold=0.5
  Switch1 : Switch  Criteria=u2 > Threshold  Threshold=0.5
  Out1 : Outport  VectorParamsAs1DForOutWhenUnconnected=off
  wires:
  Gain/1 -> Interval Test/1, Interval Test1/1
  Switch1/1 -> Add/2
  Constant/1 -> Switch1/1, Switch/1
  Constant1/1 -> Switch1/3, Switch/3
  Add/1 -> Out1/1
  Interval Test1/1 -> Switch1/2
  Switch/1 -> Add/1
  Interval Test/1 -> Switch/2
  Clock/1 -> Gain/1

== system Microgrid_W/House 4 W1/Phone_Charger/D10 ==
  Add : Sum
  Clock : Clock
  Constant : Constant
  Constant1 : Constant  Value=0
  Gain : Gain  Gain=t
  Interval Test : simulink/Logic and Bit Operations/Interval Test  IntervalClosedRight=on  uplimit=Phone_C_2_Off_a+86400*2  IntervalClosedLeft=on  lowlimit=Phone_C_2_On_a+86400*2  OutDataTypeStr=boolean
  Interval Test1 : simulink/Logic and Bit Operations/Interval Test  IntervalClosedRight=on  uplimit=Phone_C_2_Off_b+86400*2  IntervalClosedLeft=on  lowlimit=Phone_C_2_On_b+86400*2  OutDataTypeStr=boolean
  Switch : Switch  Criteria=u2 > Threshold  Threshold=0.5
  Switch1 : Switch  Criteria=u2 > Threshold  Threshold=0.5
  Out1 : Outport  VectorParamsAs1DForOutWhenUnconnected=off
  wires:
  Interval Test/1 -> Switch/2
  Switch/1 -> Add/1
  Interval Test1/1 -> Switch1/2
  Add/1 -> Out1/1
  Constant1/1 -> Switch/3, Switch1/3
  Constant/1 -> Switch/1, Switch1/1
  Switch1/1 -> Add/2
  Gain/1 -> Interval Test1/1, Interval Test/1
  Clock/1 -> Gain/1

== system Microgrid_W/House 4 W1/Phone_Charger/D11 ==
  Add : Sum
  Clock : Clock
  Constant : Constant
  Constant1 : Constant  Value=0
  Gain : Gain  Gain=t
  Interval Test : simulink/Logic and Bit Operations/Interval Test  IntervalClosedRight=on  uplimit=Phone_C_2_Off_a+86400*3  IntervalClosedLeft=on  lowlimit=Phone_C_2_On_a+86400*3  OutDataTypeStr=boolean
  Interval Test1 : simulink/Logic and Bit Operations/Interval Test  IntervalClosedRight=on  uplimit=Phone_C_2_Off_b+86400*3  IntervalClosedLeft=on  lowlimit=Phone_C_2_On_b+86400*3  OutDataTypeStr=boolean
  Switch : Switch  Criteria=u2 > Threshold  Threshold=0.5
  Switch1 : Switch  Criteria=u2 > Threshold  Threshold=0.5
  Out1 : Outport  VectorParamsAs1DForOutWhenUnconnected=off
  wires:
  Gain/1 -> Interval Test/1, Interval Test1/1
  Switch1/1 -> Add/2
  Constant/1 -> Switch1/1, Switch/1
  Constant1/1 -> Switch1/3, Switch/3
  Add/1 -> Out1/1
  Interval Test1/1 -> Switch1/2
  Switch/1 -> Add/1
  Interval Test/1 -> Switch/2
  Clock/1 -> Gain/1

== system Microgrid_W/House 4 W1/Phone_Charger/D12 ==
  Add : Sum
  Clock : Clock
  Constant : Constant
  Constant1 : Constant  Value=0
  Gain : Gain  Gain=t
  Interval Test : simulink/Logic and Bit Operations/Interval Test  IntervalClosedRight=on  uplimit=Phone_C_2_Off_a+86400*4  IntervalClosedLeft=on  lowlimit=Phone_C_2_On_a+86400*4  OutDataTypeStr=boolean
  Interval Test1 : simulink/Logic and Bit Operations/Interval Test  IntervalClosedRight=on  uplimit=Phone_C_2_Off_b+86400*4  IntervalClosedLeft=on  lowlimit=Phone_C_2_On_b+86400*4  OutDataTypeStr=boolean
  Switch : Switch  Criteria=u2 > Threshold  Threshold=0.5
  Switch1 : Switch  Criteria=u2 > Threshold  Threshold=0.5
  Out1 : Outport  VectorParamsAs1DForOutWhenUnconnected=off
  wires:
  Interval Test/1 -> Switch/2
  Switch/1 -> Add/1
  Interval Test1/1 -> Switch1/2
  Add/1 -> Out1/1
  Constant1/1 -> Switch/3, Switch1/3
  Constant/1 -> Switch/1, Switch1/1
  Switch1/1 -> Add/2
  Gain/1 -> Interval Test1/1, Interval Test/1
  Clock/1 -> Gain/1

== system Microgrid_W/House 4 W1/Phone_Charger/D13 ==
  Add : Sum
  Clock : Clock
  Constant : Constant
  Constant1 : Constant  Value=0
  Gain : Gain  Gain=t
  Interval Test : simulink/Logic and Bit Operations/Interval Test  IntervalClosedRight=on  uplimit=Phone_C_2_Off_a+86400*5  IntervalClosedLeft=on  lowlimit=Phone_C_2_On_a+86400*5  OutDataTypeStr=boolean
  Interval Test1 : simulink/Logic and Bit Operations/Interval Test  IntervalClosedRight=on  uplimit=Phone_C_2_Off_b+86400*5  IntervalClosedLeft=on  lowlimit=Phone_C_2_On_b+86400*5  OutDataTypeStr=boolean
  Switch : Switch  Criteria=u2 > Threshold  Threshold=0.5
  Switch1 : Switch  Criteria=u2 > Threshold  Threshold=0.5
  Out1 : Outport  VectorParamsAs1DForOutWhenUnconnected=off
  wires:
  Gain/1 -> Interval Test/1, Interval Test1/1
  Switch1/1 -> Add/2
  Constant/1 -> Switch1/1, Switch/1
  Constant1/1 -> Switch1/3, Switch/3
  Add/1 -> Out1/1
  Interval Test1/1 -> Switch1/2
  Switch/1 -> Add/1
  Interval Test/1 -> Switch/2
  Clock/1 -> Gain/1

== system Microgrid_W/House 4 W1/Phone_Charger/D14 ==
  Add : Sum
  Clock : Clock
  Constant : Constant
  Constant1 : Constant  Value=0
  Gain : Gain  Gain=t
  Interval Test : simulink/Logic and Bit Operations/Interval Test  IntervalClosedRight=on  uplimit=Phone_C_2_Off_a+86400*6  IntervalClosedLeft=on  lowlimit=Phone_C_2_On_a+86400*6  OutDataTypeStr=boolean
  Interval Test1 : simulink/Logic and Bit Operations/Interval Test  IntervalClosedRight=on  uplimit=Phone_C_2_Off_b+86400*6  IntervalClosedLeft=on  lowlimit=Phone_C_2_On_b+86400*6  OutDataTypeStr=boolean
  Switch : Switch  Criteria=u2 > Threshold  Threshold=0.5
  Switch1 : Switch  Criteria=u2 > Threshold  Threshold=0.5
  Out1 : Outport  VectorParamsAs1DForOutWhenUnconnected=off
  wires:
  Interval Test/1 -> Switch/2
  Switch/1 -> Add/1
  Interval Test1/1 -> Switch1/2
  Add/1 -> Out1/1
  Constant1/1 -> Switch/3, Switch1/3
  Constant/1 -> Switch/1, Switch1/1
  Switch1/1 -> Add/2
  Gain/1 -> Interval Test1/1, Interval Test/1
  Clock/1 -> Gain/1

== system Microgrid_W/House 4 W1/Phone_Charger/D15 ==
  Add : Sum
  Clock : Clock
  Constant : Constant
  Constant1 : Constant  Value=0
  Gain : Gain  Gain=t
  Interval Test : simulink/Logic and Bit Operations/Interval Test  IntervalClosedRight=on  uplimit=Phone_C_3_Off_a+86400  IntervalClosedLeft=on  lowlimit=Phone_C_3_On_a+86400  OutDataTypeStr=boolean
  Interval Test1 : simulink/Logic and Bit Operations/Interval Test  IntervalClosedRight=on  uplimit=Phone_C_3_Off_b+86400  IntervalClosedLeft=on  lowlimit=Phone_C_3_On_b+86400  OutDataTypeStr=boolean
  Switch : Switch  Criteria=u2 > Threshold  Threshold=0.5
  Switch1 : Switch  Criteria=u2 > Threshold  Threshold=0.5
  Out1 : Outport  VectorParamsAs1DForOutWhenUnconnected=off
  wires:
  Interval Test/1 -> Switch/2
  Switch/1 -> Add/1
  Interval Test1/1 -> Switch1/2
  Add/1 -> Out1/1
  Constant1/1 -> Switch/3, Switch1/3
  Constant/1 -> Switch/1, Switch1/1
  Switch1/1 -> Add/2
  Gain/1 -> Interval Test1/1, Interval Test/1
  Clock/1 -> Gain/1

== system Microgrid_W/House 4 W1/Phone_Charger/D16 ==
  Add : Sum
  Clock : Clock
  Constant : Constant
  Constant1 : Constant  Value=0
  Gain : Gain  Gain=t
  Interval Test : simulink/Logic and Bit Operations/Interval Test  IntervalClosedRight=on  uplimit=Phone_C_3_Off_a+86400*2  IntervalClosedLeft=on  lowlimit=Phone_C_3_On_a+86400*2  OutDataTypeStr=boolean
  Interval Test1 : simulink/Logic and Bit Operations/Interval Test  IntervalClosedRight=on  uplimit=Phone_C_3_Off_b+86400*2  IntervalClosedLeft=on  lowlimit=Phone_C_3_On_b+86400*2  OutDataTypeStr=boolean
  Switch : Switch  Criteria=u2 > Threshold  Threshold=0.5
  Switch1 : Switch  Criteria=u2 > Threshold  Threshold=0.5
  Out1 : Outport  VectorParamsAs1DForOutWhenUnconnected=off
  wires:
  Gain/1 -> Interval Test/1, Interval Test1/1
  Switch1/1 -> Add/2
  Constant/1 -> Switch1/1, Switch/1
  Constant1/1 -> Switch1/3, Switch/3
  Add/1 -> Out1/1
  Interval Test1/1 -> Switch1/2
  Switch/1 -> Add/1
  Interval Test/1 -> Switch/2
  Clock/1 -> Gain/1

== system Microgrid_W/House 4 W1/Phone_Charger/D17 ==
  Add : Sum
  Clock : Clock
  Constant : Constant
  Constant1 : Constant  Value=0
  Gain : Gain  Gain=t
  Interval Test : simulink/Logic and Bit Operations/Interval Test  IntervalClosedRight=on  uplimit=Phone_C_3_Off_a+86400*3  IntervalClosedLeft=on  lowlimit=Phone_C_3_On_a+86400*3  OutDataTypeStr=boolean
  Interval Test1 : simulink/Logic and Bit Operations/Interval Test  IntervalClosedRight=on  uplimit=Phone_C_3_Off_b+86400*3  IntervalClosedLeft=on  lowlimit=Phone_C_3_On_b+86400*3  OutDataTypeStr=boolean
  Switch : Switch  Criteria=u2 > Threshold  Threshold=0.5
  Switch1 : Switch  Criteria=u2 > Threshold  Threshold=0.5
  Out1 : Outport  VectorParamsAs1DForOutWhenUnconnected=off
  wires:
  Interval Test/1 -> Switch/2
  Switch/1 -> Add/1
  Interval Test1/1 -> Switch1/2
  Add/1 -> Out1/1
  Constant1/1 -> Switch/3, Switch1/3
  Constant/1 -> Switch/1, Switch1/1
  Switch1/1 -> Add/2
  Gain/1 -> Interval Test1/1, Interval Test/1
  Clock/1 -> Gain/1

== system Microgrid_W/House 4 W1/Phone_Charger/D18 ==
  Add : Sum
  Clock : Clock
  Constant : Constant
  Constant1 : Constant  Value=0
  Gain : Gain  Gain=t
  Interval Test : simulink/Logic and Bit Operations/Interval Test  IntervalClosedRight=on  uplimit=Phone_C_3_Off_a+86400*4  IntervalClosedLeft=on  lowlimit=Phone_C_3_On_a+86400*4  OutDataTypeStr=boolean
  Interval Test1 : simulink/Logic and Bit Operations/Interval Test  IntervalClosedRight=on  uplimit=Phone_C_3_Off_b+86400*4  IntervalClosedLeft=on  lowlimit=Phone_C_3_On_b+86400*4  OutDataTypeStr=boolean
  Switch : Switch  Criteria=u2 > Threshold  Threshold=0.5
  Switch1 : Switch  Criteria=u2 > Threshold  Threshold=0.5
  Out1 : Outport  VectorParamsAs1DForOutWhenUnconnected=off
  wires:
  Gain/1 -> Interval Test/1, Interval Test1/1
  Switch1/1 -> Add/2
  Constant/1 -> Switch1/1, Switch/1
  Constant1/1 -> Switch1/3, Switch/3
  Add/1 -> Out1/1
  Interval Test1/1 -> Switch1/2
  Switch/1 -> Add/1
  Interval Test/1 -> Switch/2
  Clock/1 -> Gain/1

== system Microgrid_W/House 4 W1/Phone_Charger/D19 ==
  Add : Sum
  Clock : Clock
  Constant : Constant
  Constant1 : Constant  Value=0
  Gain : Gain  Gain=t
  Interval Test : simulink/Logic and Bit Operations/Interval Test  IntervalClosedRight=on  uplimit=Phone_C_3_Off_a+86400*5  IntervalClosedLeft=on  lowlimit=Phone_C_3_On_a+86400*5  OutDataTypeStr=boolean
  Interval Test1 : simulink/Logic and Bit Operations/Interval Test  IntervalClosedRight=on  uplimit=Phone_C_3_Off_b+86400*5  IntervalClosedLeft=on  lowlimit=Phone_C_3_On_b+86400*5  OutDataTypeStr=boolean
  Switch : Switch  Criteria=u2 > Threshold  Threshold=0.5
  Switch1 : Switch  Criteria=u2 > Threshold  Threshold=0.5
  Out1 : Outport  VectorParamsAs1DForOutWhenUnconnected=off
  wires:
  Interval Test/1 -> Switch/2
  Switch/1 -> Add/1
  Interval Test1/1 -> Switch1/2
  Add/1 -> Out1/1
  Constant1/1 -> Switch/3, Switch1/3
  Constant/1 -> Switch/1, Switch1/1
  Switch1/1 -> Add/2
  Gain/1 -> Interval Test1/1, Interval Test/1
  Clock/1 -> Gain/1

== system Microgrid_W/House 4 W1/Phone_Charger/D2 ==
  Add : Sum
  Clock : Clock
  Constant : Constant
  Constant1 : Constant  Value=0
  Gain : Gain  Gain=t
  Interval Test : simulink/Logic and Bit Operations/Interval Test  IntervalClosedRight=on  uplimit=Phone_C_1_Off_a+86400  IntervalClosedLeft=on  lowlimit=Phone_C_1_On_a+86400  OutDataTypeStr=boolean
  Interval Test1 : simulink/Logic and Bit Operations/Interval Test  IntervalClosedRight=on  uplimit=Phone_C_1_Off_b+86400  IntervalClosedLeft=on  lowlimit=Phone_C_1_On_b+86400  OutDataTypeStr=boolean
  Switch : Switch  Criteria=u2 > Threshold  Threshold=0.5
  Switch1 : Switch  Criteria=u2 > Threshold  Threshold=0.5
  Out1 : Outport  VectorParamsAs1DForOutWhenUnconnected=off
  wires:
  Interval Test/1 -> Switch/2
  Switch/1 -> Add/1
  Interval Test1/1 -> Switch1/2
  Add/1 -> Out1/1
  Constant1/1 -> Switch/3, Switch1/3
  Constant/1 -> Switch/1, Switch1/1
  Switch1/1 -> Add/2
  Gain/1 -> Interval Test1/1, Interval Test/1
  Clock/1 -> Gain/1

== system Microgrid_W/House 4 W1/Phone_Charger/D20 ==
  Add : Sum
  Clock : Clock
  Constant : Constant
  Constant1 : Constant  Value=0
  Gain : Gain  Gain=t
  Interval Test : simulink/Logic and Bit Operations/Interval Test  IntervalClosedRight=on  uplimit=Phone_C_3_Off_a  IntervalClosedLeft=on  lowlimit=Phone_C_3_On_a  OutDataTypeStr=boolean
  Interval Test1 : simulink/Logic and Bit Operations/Interval Test  IntervalClosedRight=on  uplimit=Phone_C_3_Off_b  IntervalClosedLeft=on  lowlimit=Phone_C_3_On_b  OutDataTypeStr=boolean
  Switch : Switch  Criteria=u2 > Threshold  Threshold=0.5
  Switch1 : Switch  Criteria=u2 > Threshold  Threshold=0.5
  Out1 : Outport  VectorParamsAs1DForOutWhenUnconnected=off
  wires:
  Gain/1 -> Interval Test/1, Interval Test1/1
  Switch1/1 -> Add/2
  Constant/1 -> Switch1/1, Switch/1
  Constant1/1 -> Switch1/3, Switch/3
  Add/1 -> Out1/1
  Interval Test1/1 -> Switch1/2
  Switch/1 -> Add/1
  Interval Test/1 -> Switch/2
  Clock/1 -> Gain/1
